simulink model "cstr_model"  (R2025b)
settings: Solver=VariableStepAuto  StartTime=0.0  StopTime=20  RelTol=1e-3
values from neighbouring files (symbols this model uses):
  CA_in = 1.0    (= 1)    [cstr_simulation.m]
  Cp = 0.239    [cstr_simulation.m]
  dH = -50000    [cstr_simulation.m]
  E_R = 8750    [cstr_simulation.m]
  F = 100    [cstr_simulation.m]
  k0 = 7.2e10    (= 72000000000)    [cstr_simulation.m]
  rho = 1000    [cstr_simulation.m]
  T_cool = 300    [cstr_simulation.m]
  T_in = 350    [cstr_simulation.m]
  UA = 50000    [cstr_simulation.m]
  V = 1000    [cstr_simulation.m]
settings Model: Creator=Devansh Singh  LastModifiedBy=Devansh Singh

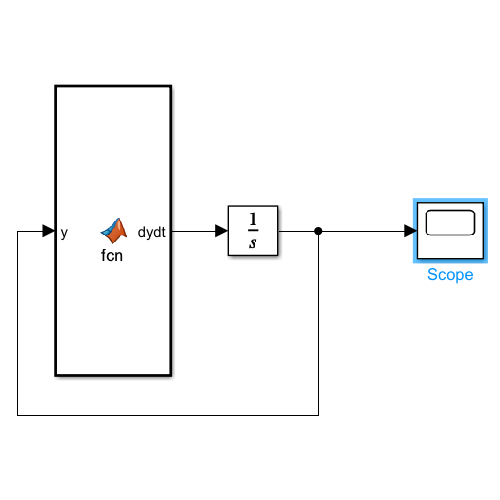
[thumbnail: Simulink's stored preview of the top-level diagram]
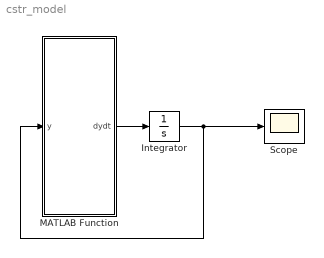
== system cstr_model ==
  Integrator : Integrator  InitialCondition=[0.1; 300]
  MATLAB Function : MATLAB Function  TreatAsAtomicUnit=on
  Scope : Scope
      settings: ActiveDisplayYMinimum=-51.607797445034372  ActiveDisplayYMaximum=464.49323645064118
  wires:
  MATLAB Function/1(dydt) -> Integrator/1
  Integrator/1 -> MATLAB Function/1(y), Scope/1

== matlab function cstr_model/MATLAB Function ==
  data: y input; F parameter; V parameter; CA_in parameter; T_in parameter; T_cool parameter; k0 parameter; E_R parameter; dH parameter; rho parameter; Cp parameter; UA parameter; dydt output
function dydt = fcn(y, F, V, CA_in, T_in, T_cool, k0, E_R, dH, rho, Cp, UA)

    % This is the exact same logic as your script!

    % Unpack variables
    CA = y(1);
    T  = y(2);

    % Arrhenius
    k = k0 * exp(-E_R / T);

    % Mass Balance
    dCAdt = (F/V)*(CA_in - CA) - k*CA;

    % Energy Balance
    dTdt = (F/V)*(T_in - T) + (-dH*k*CA)/(rho*Cp) - (UA/(rho*Cp*V))*(T - T_cool);

    % Output
    dydt = [dCAdt; dTdt];
end
